simulink model "vSimulink"  (R2017a)
settings: Solver=VariableStepAuto  StartTime=0.0  StopTime=200  RelTol=1e-3
settings Model: Creator=ITAM\vcruzg  LastModifiedBy=ITAM\vcruzg

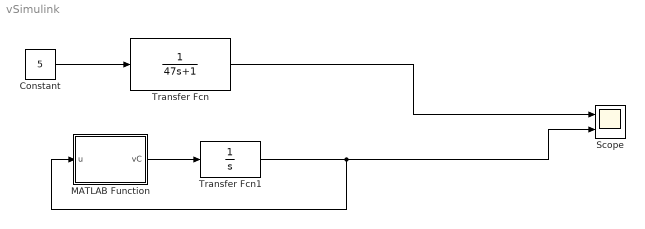
== system vSimulink ==
  Constant : Constant  Value=5
  MATLAB Function : MATLAB Function  TreatAsAtomicUnit=on
  Scope : Scope  NumInputPorts=2
  Transfer Fcn : TransferFcn  Denominator=[47 1]
  Transfer Fcn1 : TransferFcn  Denominator=[1 0]
  wires:
  Transfer Fcn/1 -> Scope/1
  Constant/1 -> Transfer Fcn/1
  MATLAB Function/1(vC) -> Transfer Fcn1/1
  Transfer Fcn1/1 -> MATLAB Function/1(u), Scope/2

== matlab function vSimulink/MATLAB Function ==
  data: u input; vC output
function vC = fcn(u)
Vin=5;
R=47000;
C=1000*10^-6;

vC = (5-u)/(R*C);
